simulink model "rtwdemo_merge"  (Simulink 6.0)
settings: Solver=FixedStepDiscrete  StartTime=0.0  StopTime=10.0  RelTol=1e-3
libraries: rtwdemowidgets x2
settings Model: CovMetricSettings=d  Creator=The MathWorks Inc.  LastModifiedBy=batserve  ExtModeAutoUpdateStatusClock=off
settings DataIOCC: SaveOutput=off  SaveTime=off  SignalLoggingName=sigsOut
settings OptimizationCC: InlineParams=on  EnforceIntegerDowncast=off  StateBitsets=on  DataBitsets=on  UseTempVars=on
settings DebuggingCC: CheckExecutionContextPreStartOutputMsg=on  CheckExecutionContextRuntimeOutputMsg=on  SolverPrmCheckMsg=none
settings RTWCC: TLCOptions=-p0 -aWarnNonSaturatedBlocks=0  GenCodeOnly=on  GenerateReport=on  RTWVerbose=off  ProcessScript=grt_make_rtw_hook  LaunchReport=on
settings CodeAppCC: ForceParamTrailComments=on  PrefixModelToSubsysFcnNames=off
settings GRTTargetCC: MatFileLogging=off

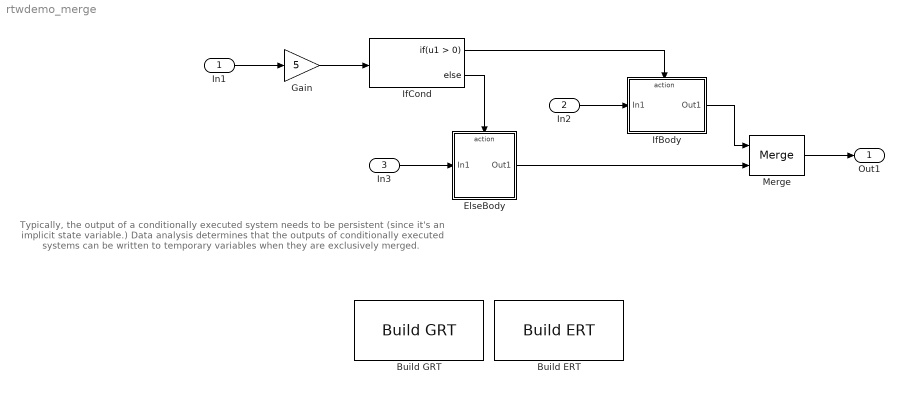
== system rtwdemo_merge ==
  note: Typically, the output of a conditionally executed system needs to be persistent (since it's an
      | implicit state variable.)  Data analysis determines that the outputs of conditionally executed
      | systems can be written to temporary variables when they are exclusively merged.
  In1 : Inport  Port=1  DataType=single  LatchInput=off
  In2 : Inport  Port=2  DataType=single  LatchInput=off
  In3 : Inport  Port=3  DataType=single  LatchInput=off
  Build ERT : rtwdemowidgets/Build ERT  attrib_overrides={}
  Build GRT : rtwdemowidgets/Build GRT  attrib_overrides={}
  ElseBody : Subsystem  TreatAsAtomicUnit=on  PropExecContextAcrossSSBoundary=on
  Gain : Gain  Gain=5  SaturateOnIntegerOverflow=on
  IfBody : Subsystem  TreatAsAtomicUnit=on  PropExecContextAcrossSSBoundary=on
  IfCond : If
  Merge : Merge
  Out1 : Outport
  wires:
  IfCond/1 -> IfBody/Action
  IfCond/2 -> ElseBody/Action
  In1/1 -> Gain/1
  In2/1 -> IfBody/1(In1)
  In3/1 -> ElseBody/1(In1)
  IfBody/1(Out1) -> Merge/1
  ElseBody/1(Out1) -> Merge/2
  Merge/1 -> Out1/1
  Gain/1 -> IfCond/1

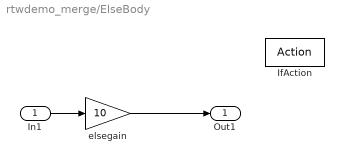
== system rtwdemo_merge/ElseBody ==
  In1 : Inport  Port=1  LatchInput=off
  IfAction : ActionPort  ActionType=else
  elsegain : Gain  Gain=10  SaturateOnIntegerOverflow=on
  Out1 : Outport
  wires:
  In1/1 -> elsegain/1
  elsegain/1 -> Out1/1

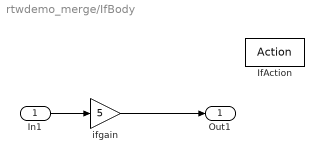
== system rtwdemo_merge/IfBody ==
  In1 : Inport  Port=1  LatchInput=off
  IfAction : ActionPort  ActionType=then
  ifgain : Gain  Gain=5  SaturateOnIntegerOverflow=on
  Out1 : Outport
  wires:
  In1/1 -> ifgain/1
  ifgain/1 -> Out1/1
